simulink model "FullModelAddANN_Final_ANN_revised"  (R2024b)
settings: Solver=ode4  StartTime=0.0  StopTime=40  FixedStep=1e-5  RelTol=1e-3
values from neighbouring files (symbols this model uses):
  Dp = 2.506338228783948e3    (= 2506.33822878)    [FullModelAddANNm_Final.m]    (also in main_opal_ann_control.m)
  Dq = 1.033099625954584    (= 1.03309962595)    [FullModelAddANNm_Final.m]    (also in main_opal_ann_control.m)
  Kp = 0.006383815167581    (= 0.00638381516758)    [FullModelAddANNm_Final.m]    (also in main_opal_ann_control.m)
  Kq = 0.076670166944346    (= 0.0766701669443)    [FullModelAddANNm_Final.m]    (also in main_opal_ann_control.m)
undefined symbols (not defined in the file or in its folder): Filter, Ls, params
libraries: neural x88, spsCurrentMeasurementLib x6, spsParallelRLCBranchLib x6, spsIGBTDiodeLib x6, spsMeanLib x6, spsSeriesRLCBranchLib x6, simulink x4, spsVoltageMeasurementLib x4, spsVariableInductorLib x3, spsVariableResistorLib x3, spsDCVoltageSourceLib x1, spsThreePhaseSourceLib x1
(part 11 of 11)

== system FullModelAddANN_Final_ANN_revised/Feed-Forward Neural Network_strength/Layer 2/Delays 1 ==
  "p{2}" : Inport  PortDimensions=16
      mask Display: e = 0.06;c1 = [120 230 180]/255;c2 = ([120 230 180]+0)/(256+128);c3 = ([120 230 180]+128)/(256+128);patch([0 1 1 0],[0 0 1 1],c1);patch([0 1 1 1-e 1-e 0+e],[0 0 1 1-e 0+e 0+e],c2);patch([0 0 1 1-e 0+e 0+e],[0 1 1 1-e 1-e 0+e],c3);plot([0 1 1 0 0],[0 0 1 1 0]);
  mux : Mux  Inputs=1
      mask Display: e = 0.06;c1 = [120 150 230]/255;c2 = ([120 150 230]+0)/383;c3 = ([120 150 230]+128)/383;patch([0 1 1 0],[0 0 1 1],c1);patch([0 1 1 1-e 1-e 0+e],[0 0 1 1-e 0+e 0+e],c2);patch([0 0 1 1-e 0+e 0+e],[0 1 1 1-e 1-e 0+e],c3);plot([0 1 1 0 0],[0 0 1 1 0]);disp('Mux')
  "pd{2,1}" : Outport
      mask Display: e = 0.06;c1 = [120 230 180]/255;c2 = ([120 230 180]+0)/(256+128);c3 = ([120 230 180]+128)/(256+128);patch([0 1 1 0],[0 0 1 1],c1);patch([0 1 1 1-e 1-e 0+e],[0 0 1 1-e 0+e 0+e],c2);patch([0 0 1 1-e 0+e 0+e],[0 1 1 1-e 1-e 0+e],c3);plot([0 1 1 0 0],[0 0 1 1 0]);
  wires:
  "p{2}"/1 -> mux/1
  mux/1 -> "pd{2,1}"/1

== system FullModelAddANN_Final_ANN_revised/Feed-Forward Neural Network_strength/Layer 2/LW{2,1} ==
  "ad{2,1}" : Inport  PortDimensions=16
      mask Display: e = 0.06;c1 = [120 230 180]/255;c2 = ([120 230 180]+0)/(256+128);c3 = ([120 230 180]+128)/(256+128);patch([0 1 1 0],[0 0 1 1],c1);patch([0 1 1 1-e 1-e 0+e],[0 0 1 1-e 0+e 0+e],c2);patch([0 0 1 1-e 0+e 0+e],[0 1 1 1-e 1-e 0+e],c3);plot([0 1 1 0 0],[0 0 1 1 0]);
  "IW{2,1}(1,:)'" : Constant  Value=[-0.1757630162071365520493060330409207381308078765869140625;0.0477511478519346554971747309537022374570369720458984375;0.36351105974383079999512347058043815195560455322265625;-0.1660388856645657329469401020105578936636447906494140625;0.318110280998365080318279751736554317176342010498046875;0.472226258270771082070638158256770111620426177978515625;0.34034223437967181524754778365604579448699951171875;0.1873321063255778129441608825800358317792415618896484375;0.08951883039914064477127197960726334713399410247802734375;-0.044959248596025604138848308366505079902708530426025390625;-0.2371556345845630964230821291494066826999187469482421875;-0.5287252851220929361630851417430676519870758056640625;-0.1944934910483313295070928461427683942019939422607421875;0.21838237504201474248333170180558227002620697021484375;-0.0269608818590906414158769877076338161714375019073486328125;-0.21792106367942964961770258014439605176448822021484375]
      mask Display: e = 0.06;c1 = [120 150 230]/255;c2 = ([120 150 230]+0)/383;c3 = ([120 150 230]+128)/383;patch([0 1 1 0],[0 0 1 1],c1);patch([0 1 1 1-e 1-e 0+e],[0 0 1 1-e 0+e 0+e],c2);patch([0 0 1 1-e 0+e 0+e],[0 1 1 1-e 1-e 0+e],c3);plot([0 1 1 0 0],[0 0 1 1 0]);disp('weights');
  "IW{2,1}(2,:)'" : Constant  Value=[-0.15881149332797728224164757193648256361484527587890625;0.1566580435625457845549846069843624718487262725830078125;0.1143600695633124886274600839897175319492816925048828125;0.286821548325872643925293914435314945876598358154296875;0.212006116860946558499989578194799832999706268310546875;0.1673353939131763390424367798914317972958087921142578125;0.1300524578706684641904445243199006654322147369384765625;-0.1577671781682230822685397697568987496197223663330078125;0.35494687042428807455252126601408235728740692138671875;-0.11632365771860235514889581054376321844756603240966796875;-0.1487174948811556263184030513002653606235980987548828125;-0.268438693679127482472068777497042901813983917236328125;-0.1468370279315009130360891731470474041998386383056640625;0.01022342334127866216031410573350513004697859287261962890625;0.25553782847197681338258234973181970417499542236328125;-0.02421920847978868696070975374823319725692272186279296875]
      mask Display: e = 0.06;c1 = [120 150 230]/255;c2 = ([120 150 230]+0)/383;c3 = ([120 150 230]+128)/383;patch([0 1 1 0],[0 0 1 1],c1);patch([0 1 1 1-e 1-e 0+e],[0 0 1 1-e 0+e 0+e],c2);patch([0 0 1 1-e 0+e 0+e],[0 1 1 1-e 1-e 0+e],c3);plot([0 1 1 0 0],[0 0 1 1 0]);disp('weights');
  Mux : Mux  Inputs=2
      mask Display: e = 0.06;c1 = [120 150 230]/255;c2 = ([120 150 230]+0)/383;c3 = ([120 150 230]+128)/383;patch([0 1 1 0],[0 0 1 1],c1);patch([0 1 1 1-e 1-e 0+e],[0 0 1 1-e 0+e 0+e],c2);patch([0 0 1 1-e 0+e 0+e],[0 1 1 1-e 1-e 0+e],c3);plot([0 1 1 0 0],[0 0 1 1 0]);disp('Mux');
  dotprod1 : neural/Weight Functions/dotprod
  dotprod2 : neural/Weight Functions/dotprod
  "lz{2,1}" : Outport
      mask Display: e = 0.06;c1 = [120 230 180]/255;c2 = ([120 230 180]+0)/(256+128);c3 = ([120 230 180]+128)/(256+128);patch([0 1 1 0],[0 0 1 1],c1);patch([0 1 1 1-e 1-e 0+e],[0 0 1 1-e 0+e 0+e],c2);patch([0 0 1 1-e 0+e 0+e],[0 1 1 1-e 1-e 0+e],c3);plot([0 1 1 0 0],[0 0 1 1 0]);
  wires:
  "IW{2,1}(1,:)'"/1 -> dotprod1/1
  "ad{2,1}"/1 -> dotprod1/2, dotprod2/2
  dotprod1/1 -> Mux/1
  "IW{2,1}(2,:)'"/1 -> dotprod2/1
  dotprod2/1 -> Mux/2
  Mux/1 -> "lz{2,1}"/1

== system FullModelAddANN_Final_ANN_revised/Inner control/Subsystem1/Subsystem1 ==
  xa : Inport
  xb : Inport  Port=2
  xc : Inport  Port=3
  Add : Sum  Inputs=+++
  Add1 : Sum
  Gain1 : Gain  Gain=-1/2
  Gain2 : Gain
  Gain3 : Gain  Gain=-1/2
  Gain4 : Gain  Gain=sqrt(3)/2
  Gain5 : Gain  Gain=-sqrt(3)/2
  Gain6 : Gain  Gain=2/3
  Gain7 : Gain  Gain=2/3
  xalpha : Outport  VectorParamsAs1DForOutWhenUnconnected=off
  xbeta : Outport  Port=2  VectorParamsAs1DForOutWhenUnconnected=off
  wires:
  xa/1 -> Gain2/1
  Gain7/1 -> xbeta/1
  Gain4/1 -> Add1/1
  Add/1 -> Gain6/1
  Gain2/1 -> Add/1
  Gain5/1 -> Add1/2
  xb/1 -> Gain1/1, Gain4/1
  Gain1/1 -> Add/2
  Gain3/1 -> Add/3
  Add1/1 -> Gain7/1
  Gain6/1 -> xalpha/1
  xc/1 -> Gain3/1, Gain5/1

== system FullModelAddANN_Final_ANN_revised/Inner control/Subsystem1/Subsystem2 ==
  xalpha : Inport
  xbeta : Inport  Port=2
  wt : Inport  Port=3
  Fcn : Fcn  Expr=cos(u(3))*u(1)+u(2)*sin(u(3))
  Fcn1 : Fcn  Expr=-sin(u(3))*u(1)+u(2)*cos(u(3))
  Mux : Mux  Inputs=3
  xd : Outport  VectorParamsAs1DForOutWhenUnconnected=off
  xq : Outport  Port=2  VectorParamsAs1DForOutWhenUnconnected=off
  wires:
  wt/1 -> Mux/3
  xalpha/1 -> Mux/1
  Fcn1/1 -> xq/1
  xbeta/1 -> Mux/2
  Fcn/1 -> xd/1
  Mux/1 -> Fcn1/1, Fcn/1

== system FullModelAddANN_Final_ANN_revised/Inner control/Subsystem3/Subsystem1 ==
  xa : Inport
  xb : Inport  Port=2
  xc : Inport  Port=3
  Add : Sum  Inputs=+++
  Add1 : Sum
  Gain1 : Gain  Gain=-1/2
  Gain2 : Gain
  Gain3 : Gain  Gain=-1/2
  Gain4 : Gain  Gain=sqrt(3)/2
  Gain5 : Gain  Gain=-sqrt(3)/2
  Gain6 : Gain  Gain=2/3
  Gain7 : Gain  Gain=2/3
  xalpha : Outport  VectorParamsAs1DForOutWhenUnconnected=off
  xbeta : Outport  Port=2  VectorParamsAs1DForOutWhenUnconnected=off
  wires:
  xc/1 -> Gain5/1, Gain3/1
  Gain6/1 -> xalpha/1
  Add1/1 -> Gain7/1
  Gain3/1 -> Add/3
  Gain1/1 -> Add/2
  xb/1 -> Gain4/1, Gain1/1
  Gain5/1 -> Add1/2
  Gain2/1 -> Add/1
  Add/1 -> Gain6/1
  Gain4/1 -> Add1/1
  Gain7/1 -> xbeta/1
  xa/1 -> Gain2/1

== system FullModelAddANN_Final_ANN_revised/Inner control/Subsystem3/Subsystem2 ==
  xalpha : Inport
  xbeta : Inport  Port=2
  wt : Inport  Port=3
  Fcn : Fcn  Expr=cos(u(3))*u(1)+u(2)*sin(u(3))
  Fcn1 : Fcn  Expr=-sin(u(3))*u(1)+u(2)*cos(u(3))
  Mux : Mux  Inputs=3
  xd : Outport  VectorParamsAs1DForOutWhenUnconnected=off
  xq : Outport  Port=2  VectorParamsAs1DForOutWhenUnconnected=off
  wires:
  wt/1 -> Mux/3
  Mux/1 -> Fcn/1, Fcn1/1
  Fcn/1 -> xd/1
  xbeta/1 -> Mux/2
  Fcn1/1 -> xq/1
  xalpha/1 -> Mux/1

== system FullModelAddANN_Final_ANN_revised/Inner control/Subsystem4/Subsystem1 ==
  xa : Inport
  xb : Inport  Port=2
  xc : Inport  Port=3
  Add : Sum  Inputs=+++
  Add1 : Sum
  Gain1 : Gain  Gain=-1/2
  Gain2 : Gain
  Gain3 : Gain  Gain=-1/2
  Gain4 : Gain  Gain=sqrt(3)/2
  Gain5 : Gain  Gain=-sqrt(3)/2
  Gain6 : Gain  Gain=2/3
  Gain7 : Gain  Gain=2/3
  xalpha : Outport  VectorParamsAs1DForOutWhenUnconnected=off
  xbeta : Outport  Port=2  VectorParamsAs1DForOutWhenUnconnected=off
  wires:
  xc/1 -> Gain5/1, Gain3/1
  Gain6/1 -> xalpha/1
  Add1/1 -> Gain7/1
  Gain3/1 -> Add/3
  Gain1/1 -> Add/2
  xb/1 -> Gain4/1, Gain1/1
  Gain5/1 -> Add1/2
  Gain2/1 -> Add/1
  Add/1 -> Gain6/1
  Gain4/1 -> Add1/1
  Gain7/1 -> xbeta/1
  xa/1 -> Gain2/1

== system FullModelAddANN_Final_ANN_revised/Inner control/Subsystem4/Subsystem2 ==
  xalpha : Inport
  xbeta : Inport  Port=2
  wt : Inport  Port=3
  Fcn : Fcn  Expr=cos(u(3))*u(1)+u(2)*sin(u(3))
  Fcn1 : Fcn  Expr=-sin(u(3))*u(1)+u(2)*cos(u(3))
  Mux : Mux  Inputs=3
  xd : Outport  VectorParamsAs1DForOutWhenUnconnected=off
  xq : Outport  Port=2  VectorParamsAs1DForOutWhenUnconnected=off
  wires:
  Mux/1 -> Fcn/1, Fcn1/1
  Fcn/1 -> xd/1
  xbeta/1 -> Mux/2
  Fcn1/1 -> xq/1
  xalpha/1 -> Mux/1
  wt/1 -> Mux/3

== system FullModelAddANN_Final_ANN_revised/Inner control/dq-abc/Subsystem2 ==
  xdq : Inport
  wt : Inport  Port=2
  Demux : Demux  Outputs=2
  Fcn2 : Fcn  Expr=u(1)*cos(u(3))-u(2)*sin(u(3))
  Fcn3 : Fcn  Expr=u(1)*sin(u(3))+u(2)*cos(u(3))
  Mux : Mux  Inputs=2
  Mux2 : Mux  Inputs=3
  xalbe : Outport  VectorParamsAs1DForOutWhenUnconnected=off
  wires:
  Mux2/1 -> Fcn2/1, Fcn3/1
  wt/1 -> Mux2/3
  xdq/1 -> Demux/1
  Demux/1 -> Mux2/1
  Demux/2 -> Mux2/2
  Fcn2/1 -> Mux/1
  Fcn3/1 -> Mux/2
  Mux/1 -> xalbe/1

== system FullModelAddANN_Final_ANN_revised/Inner control/dq-abc/Subsystem3 ==
  xalbe : Inport
  Add : Sum
  Add1 : Sum
  Demux : Demux  Outputs=2
  Gain : Gain
  Gain1 : Gain  Gain=-1/2
  Gain2 : Gain  Gain=sqrt(3)/2
  Gain3 : Gain  Gain=-1/2
  Gain4 : Gain  Gain=-sqrt(3)/2
  Mux : Mux  Inputs=3
  xabc : Outport  VectorParamsAs1DForOutWhenUnconnected=off
  wires:
  Add1/1 -> Mux/3
  Demux/1 -> Gain/1, Gain1/1, Gain3/1
  Gain1/1 -> Add/1
  Add/1 -> Mux/2
  Demux/2 -> Gain2/1, Gain4/1
  Gain3/1 -> Add1/1
  Gain4/1 -> Add1/2
  Gain/1 -> Mux/1
  Gain2/1 -> Add/2
  Mux/1 -> xabc/1
  xalbe/1 -> Demux/1

== matlab function FullModelAddANN_Final_ANN_revised/Grid impedance2/Train4 ==
  data: t input; Lg output; XR output
function [Lg, XR] = fcn(t)
    %— Tham số hệ thống ———————————————————————————————————
    Vll_rms = 110*sqrt(3);
    S_rated = 5000;
    w0      = 2*pi*50;

    %— Hồ sơ SCR, XR & thời gian bước ————————————————————
    persistent scr_vec XR_vec step_T n_scr n_XR group_T total_T
    if isempty(scr_vec)
        % scr_vec = [2, 2, 8, 12];      % các mức SCR (nhóm ngoài)
        scr_vec = [4, 4];      % các mức SCR (nhóm ngoài)
        XR_vec  = [1];     % các mức X/R (quét bên trong)
        step_T  = 20.0;        % s/bước (mỗi XR giữ step_T giây)
        n_scr   = numel(scr_vec);
        n_XR    = numel(XR_vec);

        % MỖI NHÓM = 1 giá trị SCR, quét hết n_XR bước
        group_T = step_T * n_XR;   % thời lượng cho 1 giá trị SCR
        total_T = group_T * n_scr; % thời lượng toàn bộ kịch bản
    end

    %— Bảo vệ thời gian ————————————————————————————————
    if isempty(t) || t < 0
        t_eff = 0;
    else
        t_eff = t;
    end

    %— Xác định nhóm SCR hiện tại (1..n_scr) ————————————
    g = floor(t_eff / group_T) + 1;
    if g > n_scr
        g = n_scr;                 % quá tổng thời gian -> giữ nhóm cuối
    end

    %— Thời gian nội bộ trong nhóm SCR để chọn bước XR ————
    t_in_group = t_eff - (g-1)*group_T;
    s = floor(t_in_group / step_T) + 1;   % chỉ số XR: 1..n_XR
    if s > n_XR
        s = n_XR;                          % chặn ở bước XR cuối
    end

    %— Lấy giá trị tương ứng ————————————————————————————
    scr = scr_vec(g);        % SCR theo nhóm
    XR  = XR_vec(s);         % X/R theo bước trong nhóm

    %— Tính Lg từ SCR & X/R ————————————————————————————
    Zg = Vll_rms^2 / (scr * S_rated);        % trở kháng lưới tương đương
    Xg = Zg * XR / sqrt(1 + XR^2);           % thành phần X từ X/R
    Lg = Xg / w0;                             % quy đổi ra L
end

== matlab function FullModelAddANN_Final_ANN_revised/Grid impedance2/Train1 ==
  data: Lg input; Rg output; XR input
function Rg = fcn(Lg, XR)
f0 = 50;
Rg = 2*pi*f0*Lg/XR;

== matlab function FullModelAddANN_Final_ANN_revised/Grid impedance2/Train3 ==
  data: t input; Lg output; XR output
function [Lg, XR] = fcn(t)
    %— Tham số hệ thống ———————————————————————————————————
    Vll_rms = 110*sqrt(3);
    S_rated = 5000;
    w0      = 2*pi*50;

    %— Hồ sơ SCR, XR & thời gian bước ————————————————————
    persistent scr_vec XR_vec step_T n_scr n_XR group_T total_T
    if isempty(scr_vec)
        scr_vec = [4];      % các mức SCR (nhóm ngoài)
        XR_vec  = [1, 14];     % các mức X/R (quét bên trong)
        step_T  = 20.0;        % s/bước (mỗi XR giữ step_T giây)
        n_scr   = numel(scr_vec);
        n_XR    = numel(XR_vec);

        % MỖI NHÓM = 1 giá trị SCR, quét hết n_XR bước
        group_T = step_T * n_XR;   % thời lượng cho 1 giá trị SCR
        total_T = group_T * n_scr; % thời lượng toàn bộ kịch bản
    end

    %— Bảo vệ thời gian ————————————————————————————————
    if isempty(t) || t < 0
        t_eff = 0;
    else
        t_eff = t;
    end

    %— Xác định nhóm SCR hiện tại (1..n_scr) ————————————
    g = floor(t_eff / group_T) + 1;
    if g > n_scr
        g = n_scr;                 % quá tổng thời gian -> giữ nhóm cuối
    end

    %— Thời gian nội bộ trong nhóm SCR để chọn bước XR ————
    t_in_group = t_eff - (g-1)*group_T;
    s = floor(t_in_group / step_T) + 1;   % chỉ số XR: 1..n_XR
    if s > n_XR
        s = n_XR;                          % chặn ở bước XR cuối
    end

    %— Lấy giá trị tương ứng ————————————————————————————
    scr = scr_vec(g);        % SCR theo nhóm
    XR  = XR_vec(s);         % X/R theo bước trong nhóm

    %— Tính Lg từ SCR & X/R ————————————————————————————
    Zg = Vll_rms^2 / (scr * S_rated);        % trở kháng lưới tương đương
    Xg = Zg * XR / sqrt(1 + XR^2);           % thành phần X từ X/R
    Lg = Xg / w0;                             % quy đổi ra L
end
